simulink model "gm_Copy_of_interleaver_model"  (R2020b)
settings: Solver=FixedStepDiscrete  StartTime=0.0  StopTime=30  RelTol=1e-3
libraries: hdlmdlgenlib x10, hdlsllib x6, simulink x4, commrandsrc3 x1
settings Model: Creator=wardo  LastModifiedBy=wardo
settings DataIOCC: LimitDataPoints=on  SaveOutput=off  SaveTime=off
settings OptimizationCC: BlockReduction=off  ConditionallyExecuteInputs=off  DefaultParameterBehavior=Inlined  LifeSpan=inf
settings DebuggingCC: AlgebraicLoopMsg=error  InheritedTsInSrcMsg=none  SingleTaskRateTransMsg=error  AllowSymbolicDim=off  StrictBusMsg=ErrorOnBusTreatedAsVector  SFUnexpectedBacktrackingDiag=warning  SFNoUnconditionalDefaultTransitionDiag=warning  SFExecutionAtInitializationDiag=none  ArithmeticOperatorsInVariantConditions=warning
settings HardwareCC: ProdBitPerPointer=32  ProdBitPerSizeT=32  ProdBitPerPtrDiffT=32  ProdLargestAtomicFloat=None  ProdIntDivRoundTo=Undefined  ProdEndianess=Unspecified  ProdWordSize=32  ProdHWDeviceType=ASIC/FPGA->ASIC/FPGA  ProdEqTarget=off
settings SFSimCC: SimUseLocalCustomCode=off  CustomCodeUndefinedFunction=UseInterfaceOnly
settings RTWCC: RTWUseLocalCustomCode=off
settings CodeAppCC: StateflowObjectComments=on
settings GRTTargetCC: TargetLangStandard=C89/C90 (ANSI)
settings ConfigComp: CovScope=ReferencedModels  CovMetricSettings=dw  CovSaveCumulativeToWorkspaceVar=on  CovSaveSingleToWorkspaceVar=on  CovExternalEMLEnable=off  CovSFcnEnable=off

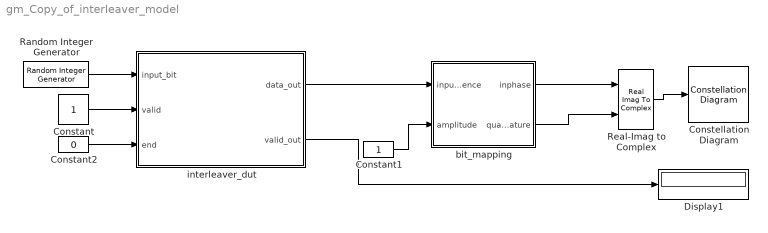
== system gm_Copy_of_interleaver_model ==
  Constant : Constant  OutDataTypeStr=boolean  SampleTime=-1
  Constant1 : Constant  OutMin=0  OutMax=5  OutDataTypeStr=fixdt(1,16)  SampleTime=-1
  Constant2 : Constant  Value=0  OutDataTypeStr=boolean  SampleTime=-1
  Constellation Diagram : ConstellationDiagram
  Display1 : Display
  Random Integer Generator : commrandsrc3/Random Integer Generator  SetSize=2  SeedSource=Auto  Seed=0  SampleTime=1  SamplesPerFrame=1  OutputDataType=boolean  SimulateUsing=Interpreted execution
  Real-Imag to Complex : RealImagToComplex
  bit_mapping : Subsystem
  interleaver_dut : Subsystem
  wires:
  Constant2/1 -> interleaver_dut/3(end)
  interleaver_dut/1(data_out) -> bit_mapping/1(input_sequence)
  Constant1/1 -> bit_mapping/2(amplitude)
  bit_mapping/2(quadrature) -> Real-Imag to Complex/2
  bit_mapping/1(inphase) -> Real-Imag to Complex/1
  Real-Imag to Complex/1 -> Constellation Diagram/1
  interleaver_dut/2(valid_out) -> Display1/1
  Constant/1 -> interleaver_dut/2(valid)
  Random Integer Generator/1 -> interleaver_dut/1(input_bit)

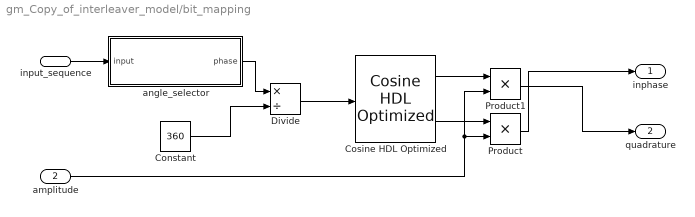
== system gm_Copy_of_interleaver_model/bit_mapping ==
  input_sequence : Inport
  amplitude : Inport  Port=2
  Constant : Constant  Value=360  OutDataTypeStr=fixdt(0,9,0)  SampleTime=-1
  Cosine HDL Optimized : hdlsllib/Lookup Tables/Cosine HDL Optimized  OutputFormula=sin(2*pi*u) and cos(2*pi*u)  NumDataPoints=32  TableDataTypeStr=fixdt(1,16,15)  SimulateLUTROMDelay=off
      settings: SourceProductBaseCode=SL
  Divide : Product  Inputs=*/  OutMin=0  OutMax=1  OutDataTypeStr=fixdt(1,16,14)  RndMeth=Zero  SaturateOnIntegerOverflow=on
  Product : Product
  Product1 : Product
  angle_selector : MATLAB Function  TreatAsAtomicUnit=on
  inphase : Outport  VectorParamsAs1DForOutWhenUnconnected=off
  quadrature : Outport  Port=2  VectorParamsAs1DForOutWhenUnconnected=off
  wires:
  Constant/1 -> Divide/2
  angle_selector/1(phase) -> Divide/1
  Divide/1 -> Cosine HDL Optimized/1
  Cosine HDL Optimized/1 -> Product1/1
  Cosine HDL Optimized/2 -> Product/1
  amplitude/1 -> Product/2, Product1/2
  input_sequence/1 -> angle_selector/1(input)
  Product1/1 -> quadrature/1
  Product/1 -> inphase/1

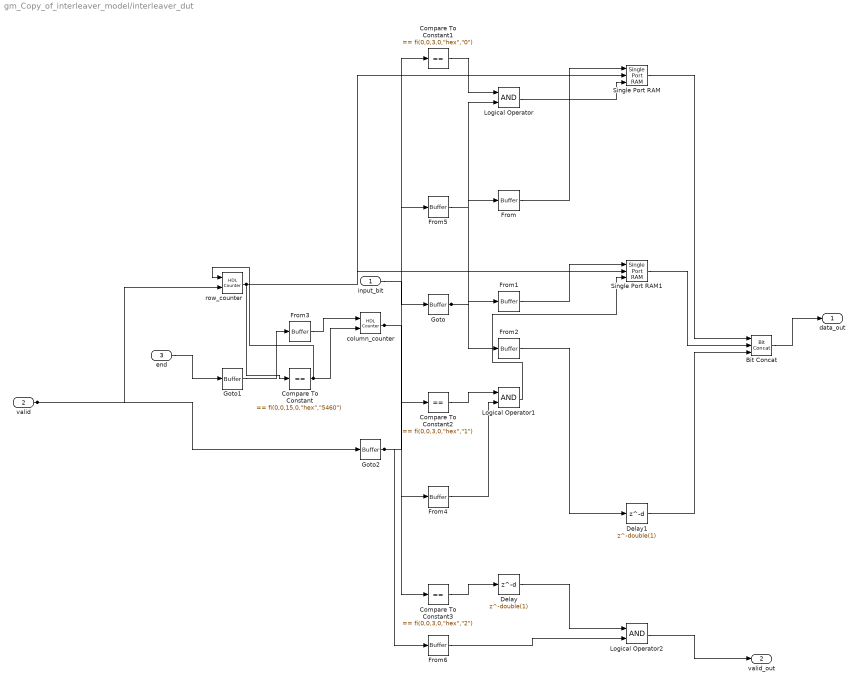
== system gm_Copy_of_interleaver_model/interleaver_dut ==
  input_bit : Inport  OutDataTypeStr=boolean  PortDimensions=1  SampleTime=1
  valid : Inport  Port=2  OutDataTypeStr=boolean  PortDimensions=1  SampleTime=1
  end : Inport  Port=3  OutDataTypeStr=boolean  PortDimensions=1  SampleTime=1
  Bit Concat : hdlsllib/Logic and Bit Operations/Bit Concat  numInputs=3
  Compare To Constant : simulink/Logic and Bit Operations/Compare To Constant  relop===  const="fi(0,0,15,0,\"hex\",\"5460\")"  OutDataTypeStr=boolean
  Compare To Constant1 : simulink/Logic and Bit Operations/Compare To Constant  relop===  const="fi(0,0,3,0,\"hex\",\"0\")"  OutDataTypeStr=boolean
  Compare To Constant2 : simulink/Logic and Bit Operations/Compare To Constant  relop===  const="fi(0,0,3,0,\"hex\",\"1\")"  OutDataTypeStr=boolean
  Compare To Constant3 : simulink/Logic and Bit Operations/Compare To Constant  relop===  const="fi(0,0,3,0,\"hex\",\"2\")"  OutDataTypeStr=boolean
  Delay : Delay  DelayLength=double(1)  InitialCondition=0  SampleTime=1
  Delay1 : Delay  DelayLength=double(1)  InitialCondition=0  SampleTime=1
  From{,1..6} (7 alike) : hdlmdlgenlib/Buffer
      settings: SourceProductBaseCode=SL
  Goto : hdlmdlgenlib/Buffer
      settings: SourceProductBaseCode=SL
  Goto1 : hdlmdlgenlib/Buffer
      settings: SourceProductBaseCode=SL
  Goto2 : hdlmdlgenlib/Buffer
      settings: SourceProductBaseCode=SL
  Logical Operator : Logic  AllPortsSameDT=off  OutDataTypeStr=boolean  SampleTime=1
  Logical Operator1 : Logic  AllPortsSameDT=off  OutDataTypeStr=boolean  SampleTime=1
  Logical Operator2 : Logic  AllPortsSameDT=off  OutDataTypeStr=boolean  SampleTime=1
  Single Port RAM : hdlsllib/HDL RAMs/Single Port RAM  ram_size=15  dout_type=New data
      settings: SourceProductBaseCode=SL
  Single Port RAM1 : hdlsllib/HDL RAMs/Single Port RAM  ram_size=15  dout_type=New data
      settings: SourceProductBaseCode=SL
  column_counter : hdlsllib/Sources/HDL Counter  CountType=Count limited  CountInit=double(0)  CountStep=double(1)  CountMax=double(2)  CountFromType=Initial value  CountFrom=double(0)  CountResetPort=on  CountLoadPort=off  CountEnbPort=on  CountDirPort=off  CountDataType=Unsigned  CountWordLen=3  CountFracLen=0  CountSampTime=1
  row_counter : hdlsllib/Sources/HDL Counter  CountType=Count limited  CountInit=double(1)  CountStep=double(1)  CountMax=double(21600)  CountFromType=Initial value  CountFrom=double(1)  CountResetPort=on  CountLoadPort=off  CountEnbPort=on  CountDirPort=off  CountDataType=Unsigned  CountWordLen=15  CountFracLen=0  CountSampTime=1
  data_out : Outport  VectorParamsAs1DForOutWhenUnconnected=off
  valid_out : Outport  Port=2  VectorParamsAs1DForOutWhenUnconnected=off
  wires:
  input_bit/1 -> Goto/1
  valid/1 -> row_counter/2, Goto2/1
  end/1 -> Goto1/1
  Bit Concat/1 -> data_out/1
  Compare To Constant/1 -> row_counter/1, column_counter/2
  Compare To Constant1/1 -> Logical Operator/1
  Compare To Constant2/1 -> Logical Operator1/1
  Compare To Constant3/1 -> Delay/1
  Delay/1 -> Logical Operator2/1
  Delay1/1 -> Bit Concat/3
  From/1 -> Single Port RAM/1
  From1/1 -> Single Port RAM1/1
  From2/1 -> Delay1/1
  From3/1 -> column_counter/1
  From4/1 -> Logical Operator1/2
  From5/1 -> Logical Operator/2
  From6/1 -> Logical Operator2/2
  Logical Operator/1 -> Single Port RAM/3
  Logical Operator1/1 -> Single Port RAM1/3
  Logical Operator2/1 -> valid_out/1
  Single Port RAM/1 -> Bit Concat/1
  Single Port RAM1/1 -> Bit Concat/2
  column_counter/1 -> Compare To Constant3/1, Compare To Constant2/1, Compare To Constant1/1
  row_counter/1 -> Compare To Constant/1, Single Port RAM/2, Single Port RAM1/2
  Goto/1 -> From2/1, From1/1, From/1
  Goto1/1 -> From3/1
  Goto2/1 -> From6/1, From5/1, From4/1

== matlab function gm_Copy_of_interleaver_model/bit_mapping/angle_selector ==
  settings: fimath=fimath('RoundingMethod', 'Floor','OverflowAction', 'Wrap','ProductMode', 'FullPrecision', 'SumMode', 'FullPrecision')
  data: input input; phase output
function phase = phase_selector(input)
%#codegen
% Receives a bit sequence and returns the angle in radians of the
% corresponding 8-psk constellation symbol. Gray encoding is used as stated
% in the DVB-S2 standard.
    tmp = 0; % Start at phase 0
    if(input == 1)
        tmp=0;
    elseif(input == 0)
        tmp=45;
    elseif(input == 4)
        tmp=90;
    elseif(input == 6)
        tmp=135;
    elseif(input == 2)
        tmp=180;
    elseif(input == 3)
        tmp=225;
    elseif(input == 7)
        tmp=270;
    elseif(input == 5)
        tmp=315;
    end
    % 9 bits necessary to represent 360 degrees.
    phase = fi(tmp, 0, 23, 14, hdlfimath);
